simulink model "OpenLoopFirstOrderSystemWithVariousGain"  (R2021a)
settings: Solver=VariableStepAuto  StartTime=0.0  StopTime=10.0  RelTol=1e-3
settings Model: Creator=soumy  LastModifiedBy=soumy

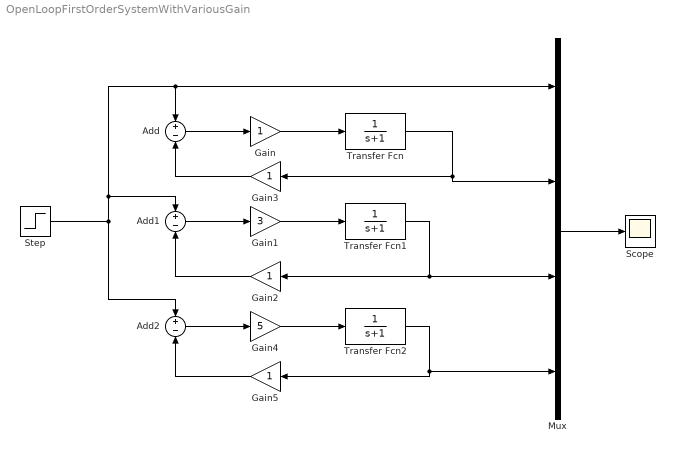
== system OpenLoopFirstOrderSystemWithVariousGain ==
  Add : Sum  Inputs=+-
  Add1 : Sum  Inputs=+-
  Add2 : Sum  Inputs=+-
  Gain{,2..3,5} (4 alike) : Gain
  Gain1 : Gain  Gain=3
  Gain4 : Gain  Gain=5
  Mux : Mux
  Scope : Scope
  Step : Step  SampleTime=0
  Transfer Fcn : TransferFcn  Denominator=[1 1]
  Transfer Fcn1 : TransferFcn  Denominator=[1 1]
  Transfer Fcn2 : TransferFcn  Denominator=[1 1]
  wires:
  Gain/1 -> Transfer Fcn/1
  Mux/1 -> Scope/1
  Add/1 -> Gain/1
  Transfer Fcn/1 -> Mux/2, Gain3/1
  Gain3/1 -> Add/2
  Add1/1 -> Gain1/1
  Gain1/1 -> Transfer Fcn1/1
  Transfer Fcn1/1 -> Gain2/1, Mux/3
  Gain2/1 -> Add1/2
  Add2/1 -> Gain4/1
  Gain4/1 -> Transfer Fcn2/1
  Transfer Fcn2/1 -> Gain5/1, Mux/4
  Gain5/1 -> Add2/2
  Step/1 -> Add2/1, Add1/1, Add/1, Mux/1
